simulink subsystem "Stanley_Controller"  (R2024b)
settings: Solver=VariableStepAuto  StartTime=0.0  StopTime=10.0  RelTol=1e-3
libraries: drivingvehiclecontroller x1
settings Model: Creator=Tong  LastModifiedBy=Tong

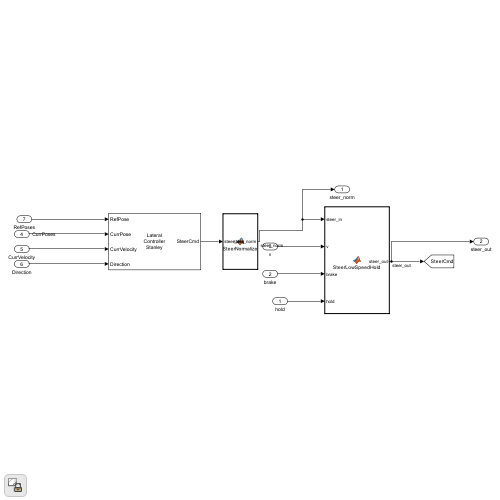
[thumbnail: Simulink's stored preview of the top-level diagram]
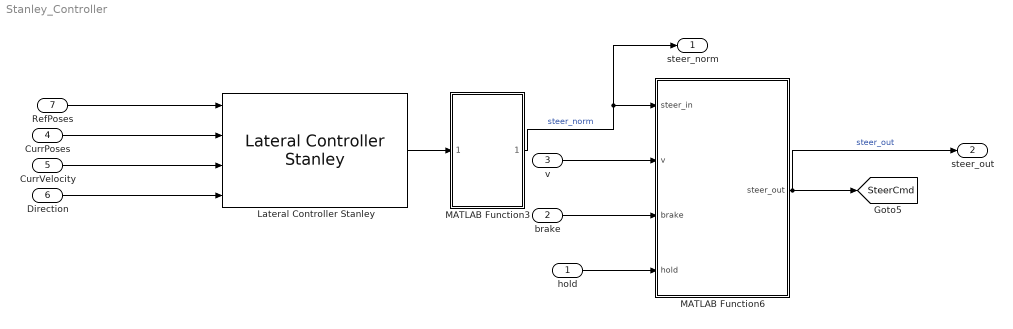
== system Stanley_Controller ==
  hold : Inport
  brake : Inport  Port=2
  v : Inport  Port=3
  CurrPoses : Inport  Port=4
  CurrVelocity : Inport  Port=5
  Direction : Inport  Port=6
  RefPoses : Inport  Port=7
  Lateral Controller Stanley : drivingvehiclecontroller/Lateral Controller Stanley  ModelType=Kinematic bicycle model  PositionGainF=2.5  PositionGainR=2.5  YawRateGain=0.2  DelayGain=0.2  VehicleMass=1575  Lf=1.2  Lr=1.6  TireStiffness=19000  Wheelbase=2.6  MaxSteeringAngle=35
  MATLAB Function3 : MATLAB Function  TreatAsAtomicUnit=on
  MATLAB Function6 : MATLAB Function  TreatAsAtomicUnit=on
  steer_norm : Outport
  steer_out : Outport  Port=2
  tag scope: SteerCmd=global
  wires:
  v/1 -> MATLAB Function6/2(v)
  brake/1 -> MATLAB Function6/3(brake)
  MATLAB Function3/1(steer_norm) -> MATLAB Function6/1(steer_in), steer_norm/1  "steer_norm"
  MATLAB Function6/1(steer_out) -> [SteerCmd], steer_out/1  "steer_out"
  Lateral Controller Stanley/1 -> MATLAB Function3/1(steer_deg)
  Direction/1 -> Lateral Controller Stanley/4
  RefPoses/1 -> Lateral Controller Stanley/1
  CurrPoses/1 -> Lateral Controller Stanley/2
  CurrVelocity/1 -> Lateral Controller Stanley/3
  hold/1 -> MATLAB Function6/4(hold)

== matlab function Stanley_Controller/MATLAB Function3 ==
  data: steer_deg input; steer_norm output
function steer_norm = SteerNormalize(steer_deg)
%#codegen
MaxSteerDeg = 35;  % 要与你Stanley块里设置一致
steer_norm = steer_deg / MaxSteerDeg;

% 限幅到[-1,1]
if steer_norm > 1
    steer_norm = 1;
elseif steer_norm < -1
    steer_norm = -1;
end
end

== matlab function Stanley_Controller/MATLAB Function6 ==
  settings: updateMethod=DISCRETE
  data: steer_in input; steer_out output; v input; brake input; hold input
% function steer_out = SteerLowSpeedHold(steer_in, v)
% %#codegen
% persistent last
% if isempty(last), last = 0; end
% 
% if v < 0.5
%     steer_out = last;   % 或改成 0 更保守
% else
%     steer_out = steer_in;
%     last = steer_in;
% end
% 
% if steer_out > 1, steer_out = 1; end
% if steer_out < -1, steer_out = -1; end
% end


function steer_out = SteerLowSpeedHold(steer_in, v, brake, hold)
%#codegen
persistent last
if isempty(last), last = 0; end

% 低速/强制停车保持/强刹时：冻结或归零转向
% if hold || (v < 0.5) || (brake > 0.7)
if hold || (v < 2)
    steer_out = 0;     % 更平滑；你也可以改成 0 更保守
else
    steer_out = steer_in;
    last = steer_in;
end

% 限幅
if steer_out > 1, steer_out = 1; end
if steer_out < -1, steer_out = -1; end
end
